simulink model "Handling_1"  (R2025b)
settings: Solver=VariableStepAuto  StartTime=0.0  StopTime=10.0  RelTol=1e-3
libraries: opcualib x1
settings Model: Creator=guilh  LastModifiedBy=guilh

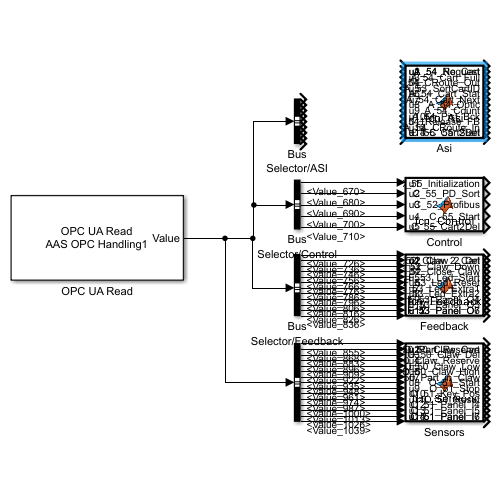
[thumbnail: Simulink's stored preview of the top-level diagram]
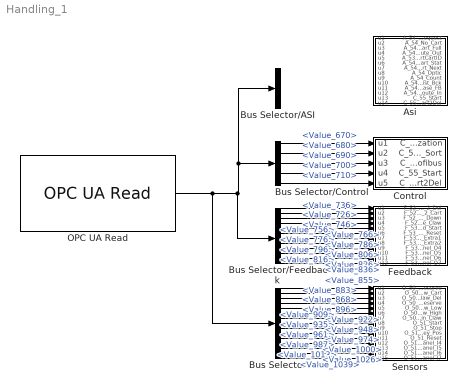
== system Handling_1 ==
  Asi : MATLAB Function  TreatAsAtomicUnit=on
  Bus Selector : BusSelector  OutputSignals=Value_855,Value_868,Value_883,Value_896,Value_909,Value_922,Value_935,Value_948,Value_961,Value_974,Value_987,Value_1000,Value_1013,Value_1026,Value_1039
  Bus Selector/ASI : BusSelector  OutputSignals=Value_574,Value_584,Value_594,Value_604,Value_614,Value_624,Value_634,Value_644,Value_654
  Bus Selector/Control : BusSelector  OutputSignals=Value_670,Value_680,Value_690,Value_700,Value_710
  Bus Selector/Feedback : BusSelector  OutputSignals=Value_726,Value_736,Value_746,Value_756,Value_766,Value_776,Value_786,Value_796,Value_806,Value_816,Value_826,Value_836
  Control : MATLAB Function  TreatAsAtomicUnit=on
  Feedback : MATLAB Function  TreatAsAtomicUnit=on
  OPC UA Read : opcualib/OPC UA Read  SelectedServer=AAS OPC Handling1  ServerList=AAS OPC Handling1  NodeList={ '1', 'Value', '6', '574', '1'; '2', 'Value', '6', '584', '1'; '3', 'Value', '6', '594', '1'; '4', 'Value', '6', '604', '1'; '5', 'Value', '6', '614', '1'; '6', 'Value', '6', '624', '1'; '7', 'Value', '6', '634', '1'; '8', 'Value', '6', '644', '1'; '9', 'Value', '6', '654', '1'; '10', 'Value', '6', '670', '1'; '11', 'Value', '6', '680', '1'; '12', 'Value', '6', '690', '1'; '13', 'Value', '6', '700', '1'; '14', 'Value', '6', '710', '1'; '15', 'Value', '6', '726', '1'; '16', 'Value', '6', '736', '1'; '17', 'Value', '6', '746', '1'; '18', 'Value', '6', '756', '1'; '19', 'Value', '6', '766', '1'; '20', 'Value', '6', '776', '1'; '21', 'Value', '6', '786', '1'; '22', 'Value', '6', '796', '1'; '23', 'Value', '6', '806', '1'; '24', 'Value', '6', '816', '1'; '25', 'Value', '6', '826', '1'; '26', 'Value', '6', '836', '1'; '27', 'Value', '6', '855', '1'; '28', 'Value', '6', '868', '1'; '29', 'Value', '6', '883', '1'; '30', 'Value', '6', '896', '1'; '31', 'Value', '6', '909', '1'; '32', 'Value', '6', '922', '1'; '33', 'Value', '6', '935', '1'; '34', 'Value', '6', '948', '1'; '35', 'Value', '6', '961', '1'; '36', 'Value', '6', '974', '1'; '37', 'Value', '6', '987', '1'; '38', 'Value', '6', '1000', '1'; '39', 'Value', '6', '1013', '1'; '40', 'Value', '6', '1026', '1'; '41', 'Value', '6', '1039', '1' }  ShowQualityPort=off  ShowTimestampPort=off  ShowTimestampPortAs=Seconds since start  SampleTime=-1
  Sensors : MATLAB Function  TreatAsAtomicUnit=on
  wires:
  OPC UA Read/1 -> Bus Selector/1, Bus Selector/Feedback/1, Bus Selector/Control/1, Bus Selector/ASI/1
  Bus Selector/Control/1 -> Control/1(u1)  "<Value_670>"
  Bus Selector/Control/2 -> Control/2(u2)  "<Value_680>"
  Bus Selector/Control/3 -> Control/3(u3)  "<Value_690>"
  Bus Selector/Control/4 -> Control/4(u4)  "<Value_700>"
  Bus Selector/Control/5 -> Control/5(u5)  "<Value_710>"
  Bus Selector/Feedback/1 -> Feedback/1(u1)  "<Value_726>"
  Bus Selector/Feedback/2 -> Feedback/2(u2)  "<Value_736>"
  Bus Selector/Feedback/3 -> Feedback/3(u3)  "<Value_746>"
  Bus Selector/Feedback/4 -> Feedback/4(u4)  "<Value_756>"
  Bus Selector/Feedback/5 -> Feedback/5(u5)  "<Value_766>"
  Bus Selector/Feedback/6 -> Feedback/6(u6)  "<Value_776>"
  Bus Selector/Feedback/7 -> Feedback/7(u7)  "<Value_786>"
  Bus Selector/Feedback/8 -> Feedback/8(u8)  "<Value_796>"
  Bus Selector/Feedback/9 -> Feedback/9(u9)  "<Value_806>"
  Bus Selector/Feedback/10 -> Feedback/10(u10)  "<Value_816>"
  Bus Selector/Feedback/11 -> Feedback/11(u11)  "<Value_826>"
  Bus Selector/Feedback/12 -> Feedback/12(u12)  "<Value_836>"
  Bus Selector/1 -> Sensors/1(u1)  "<Value_855>"
  Bus Selector/2 -> Sensors/2(u2)  "<Value_868>"
  Bus Selector/3 -> Sensors/3(u3)  "<Value_883>"
  Bus Selector/4 -> Sensors/4(u4)  "<Value_896>"
  Bus Selector/5 -> Sensors/5(u5)  "<Value_909>"
  Bus Selector/6 -> Sensors/6(u6)  "<Value_922>"
  Bus Selector/7 -> Sensors/7(u7)  "<Value_935>"
  Bus Selector/8 -> Sensors/8(u8)  "<Value_948>"
  Bus Selector/9 -> Sensors/9(u9)  "<Value_961>"
  Bus Selector/10 -> Sensors/10(u10)  "<Value_974>"
  Bus Selector/11 -> Sensors/11(u11)  "<Value_987>"
  Bus Selector/12 -> Sensors/12(u12)  "<Value_1000>"
  Bus Selector/13 -> Sensors/13(u13)  "<Value_1013>"
  Bus Selector/14 -> Sensors/14(u14)  "<Value_1026>"
  Bus Selector/15 -> Sensors/15(u15)  "<Value_1039>"

== matlab function Handling_1/Sensors ==
  data: u1 input; O_50_Part_Reserve output; u2 input; u3 input; u4 input; u5 input; u6 input; u7 input; u8 input; u9 input; u10 input; u11 input; u12 input; u13 input; u14 input; u15 input; O_50_Claw_Cart output; O_50_Claw_Del output; O_50_Claw_Reserve output; O_50_Claw_Low output; O_50_Claw_High output; O_50_Part_in_Claw output; O_51_Start output; O_51_Stop output; O_51_Key_Pos output; O_51_Reset output; O_51_Panel_I4 output; O_51_Panel_I5 output; O_51_Panel_I6 output; O_51_Panel_I7 output
function [O_50_Part_Reserve,O_50_Claw_Cart,O_50_Claw_Del,...
    O_50_Claw_Reserve,O_50_Claw_Low,O_50_Claw_High,O_50_Part_in_Claw,...
    O_51_Start,O_51_Stop,O_51_Key_Pos,O_51_Reset,O_51_Panel_I4,...
    O_51_Panel_I5,O_51_Panel_I6,O_51_Panel_I7] = fcn_Sensors(u1,u2,u3,u4,...
    u5,u6,u7,u8,u9,u10,u11,u12,u13,u14,u15)

O_50_Part_Reserve = u1;
O_50_Claw_Cart = u2;
O_50_Claw_Del = u3;
O_50_Claw_Reserve = u4;
O_50_Claw_Low = u5;
O_50_Claw_High = u6;
O_50_Part_in_Claw = u7;
O_51_Start = u8;
O_51_Stop = u9;
O_51_Key_Pos = u10;
O_51_Reset = u11;
O_51_Panel_I4 = u12;
O_51_Panel_I5 = u13;
O_51_Panel_I6 = u14;
O_51_Panel_I7 = u15;

== matlab function Handling_1/Control ==
  data: u1 input; C_55_Initialization output; u2 input; u3 input; u4 input; u5 input; C_55_PD_Sort output; C_52_Profibus output; C_55_Start output; C_55_Cart2Del output
function [C_55_Initialization,C_55_PD_Sort,C_52_Profibus,...
    C_55_Start,C_55_Cart2Del] = fcn_Control(u1,u2,u3,u4,u5)

C_55_Initialization = u1;
C_55_PD_Sort = u2;
C_52_Profibus = u3;
C_55_Start = u4;
C_55_Cart2Del = u5;

== matlab function Handling_1/Asi ==
  data: u1 input; u2 input; u3 input; u4 input; u5 input; u6 input; u7 input; u8 input; u9 input; u10 input; u11 input; u12 input; u13 input; u14 input; A_54_Request output; A_54_No_Cart output; A_54_Cart_Full output; A_54_CRoute_Out output; A_53_SortCartID output; A_54_Cart_Stat output; A_54_Cart_Next output; A_54_Optic output; A_54_Count output; A_54_Pist_Bck output; A_54_Release_FB output; A_54_CRoute_In output; C_55_Start output; C_55_Cart2Del output
function [A_54_Request, A_54_No_Cart, A_54_Cart_Full, A_54_CRoute_Out, ...
A_53_SortCartID, A_54_Cart_Stat, A_54_Cart_Next, A_54_Optic, A_54_Count,...
A_54_Pist_Bck, A_54_Release_FB, A_54_CRoute_In, C_55_Start, C_55_Cart2Del]...
= fcn_Asi(u1,u2,u3,u4,u5,u6,u7,u8,u9,u10,u11,u12,u13,u14)

A_54_Request = u1;
A_54_No_Cart = u2;
A_54_Cart_Full = u3;
A_54_CRoute_Out = u4;
A_53_SortCartID = u5;
A_54_Cart_Stat = u6;
A_54_Cart_Next = u7;
A_54_Optic = u8;
A_54_Count = u9;
A_54_Pist_Bck = u10;
A_54_Release_FB = u11;
A_54_CRoute_In = u12;
C_55_Start = u13;
C_55_Cart2Del = u14;

== matlab function Handling_1/Feedback ==
  data: u1 input; F_52_Claw_2_Del output; u2 input; u3 input; u4 input; u5 input; u6 input; u7 input; u8 input; u9 input; u10 input; u11 input; u12 input; F_52_Claw_2_Cart output; F_52_Claw_Down output; F_52_Close_Claw output; F_53_Led_Start output; F_53_Led_Reset output; F_53_Led_Extra1 output; F_53_Led_Extra2 output; F_53_Panel_O4 output; F_53_Panel_O5 output; F_53_Panel_O6 output; F_53_Panel_O7 output
function [F_52_Claw_2_Del,F_52_Claw_2_Cart,F_52_Claw_Down,...
    F_52_Close_Claw,F_53_Led_Start,F_53_Led_Reset,F_53_Led_Extra1,...
    F_53_Led_Extra2,F_53_Panel_O4,F_53_Panel_O5,F_53_Panel_O6,...
    F_53_Panel_O7] = fcn_Feedback(u1,u2,u3,u4,u5,u6,u7,u8,u9,u10,u11,u12)

F_52_Claw_2_Del = u1;
F_52_Claw_2_Cart = u2;
F_52_Claw_Down = u3;
F_52_Close_Claw = u4;
F_53_Led_Start = u5;
F_53_Led_Reset = u6;
F_53_Led_Extra1 = u7;
F_53_Led_Extra2 = u8;
F_53_Panel_O4 = u9;
F_53_Panel_O5 = u10;
F_53_Panel_O6 = u11;
F_53_Panel_O7 = u12;
